simulink model "six_plus_six_AcmsteeringV09_main"  (R2014a)
settings: Solver=FixedStepDiscrete  StartTime=0.0  StopTime=10.0  FixedStep=0.0005  RelTol=1e-3
InitFcn:
  | Veh_Par_wxt
values from neighbouring files (symbols this model uses):
  acc_spdctl = [0 100]    [Veh_Par_wxt.m]
  ag_thr = ecucoder_cal(ag_thr)    [Veh_Par_wxt.m]
  B = 1.8    [Veh_Par_wxt.m]
  bra_em = 100    [Veh_Par_wxt.m]
  bra_pre_gz2 = 100/3    (= 33.3333333333)    [Veh_Par_wxt.m]
  bra_pre_gz34 = 10/3    (= 3.33333333333)    [Veh_Par_wxt.m]
  bra_pre_yd = 10/2    (= 5)    [Veh_Par_wxt.m]
  brakepre_dem_data = [0 1 2 3 4 5 6 7 8 9 10]    [Veh_Par_wxt.m]
  brakeTrq_dem_data = [0 125 251 376 502 627 753 878 1004 1129 1255]    [Veh_Par_wxt.m]
  bratrq_max = 4*1255    (= 5020)    [Veh_Par_wxt.m]
  eff_tran = 0.9    [Veh_Par_wxt.m]
  ESP_switch = ecucoder_cal(ESP_switch)    [Veh_Par_wxt.m]
  G = Mass*g    (= 15696)    [Veh_Par_wxt.m]
  kd1 = ecucoder_cal(kd1)    [Veh_Par_wxt.m]
  kd2 = 0    [Veh_Par_wxt.m]
  ki1 = ecucoder_cal(ki1)    [Veh_Par_wxt.m]
  ki2 = 1    [Veh_Par_wxt.m]
  kp1 = ecucoder_cal(kp1)    [Veh_Par_wxt.m]
  kp2 = 300    [Veh_Par_wxt.m]
  L = L1+L2    (= 2.9)    [Veh_Par_wxt.m]
  premax = 100    [Veh_Par_wxt.m]
  Radius = 0.4572/2    (= 0.2286)    [Veh_Par_wxt.m]
  RC_switch = ecucoder_cal(RC_switch)    [Veh_Par_wxt.m]
  s_opt_yi = 0.15    [Veh_Par_wxt.m]
  s_opt_zhuan = 0.8    [Veh_Par_wxt.m]
  s_opt_zhuan_add = 0.05    [Veh_Par_wxt.m]
  s_opt_zhuan_table = [0.8 0.8 0.3 0.3]    [Veh_Par_wxt.m]
  spd_map_mot = [0 499.85 999.79 1500 2000 2500 3000 3500 4000 4500 4999.8 5999.8]    [Veh_Par_wxt.m]
  spd_spdctl = [0 500]    [Veh_Par_wxt.m]
  speed_thr_park = 5/3.6/Radius*tras_ratio*30/pi    (= 464.143899364)    [Veh_Par_wxt.m]
  TCS_switch = ecucoder_cal(TCS_switch)    [Veh_Par_wxt.m]
  tras_ratio = 8    [Veh_Par_wxt.m]
  trq_map_mot = [70.5 70.012 71.154 65.797 53.917 45.159 38.073 32.685 27.48 17.133 14.949 10.07]    [Veh_Par_wxt.m]
  trqmax_yd = 70.5    [Veh_Par_wxt.m]
  trqmax_zx = 70.5    [Veh_Par_wxt.m]
  trqmaxneg = -70.5    [Veh_Par_wxt.m]
  v_gain = 0.9    [Veh_Par_wxt.m]
  v_table = [0 5 20 100]    [Veh_Par_wxt.m]
  v_thr_park = 5    [Veh_Par_wxt.m]
  zhidong_bianmazhi = [-140000 750000]    [Veh_Par_wxt.m]
  zhidong_down = -140000    [Veh_Par_wxt.m]
  zhidong_up = 750000    [Veh_Par_wxt.m]
  zhidong_youmen = [0 100]    [Veh_Par_wxt.m]
  zhuanxiang_bianmazhi = [-400000 0 400000]    [Veh_Par_wxt.m]
  zhuanxiang_down = -400000    [Veh_Par_wxt.m]
  zhuanxiang_up = 400000    [Veh_Par_wxt.m]
  zhuanxiang_youmen = [-100 0 100]    [Veh_Par_wxt.m]
undefined symbols (not defined in the file or in its folder): ecucoder_acal, guzhang_lf, guzhang_lm, guzhang_lr, guzhang_rf, guzhang_rm, guzhang_rr, myFIS
libraries: simulink x979, ec5744lib x59, fuzblock x2
(part 17 of 26)

== system six_plus_six_AcmsteeringV09_main/Data_input/MCU0_3/MCU0/MCU0_HighVol_Sub ==
  In1 : Inport
  Out1 : Outport
  wires:
  In1/1 -> Out1/1

== system six_plus_six_AcmsteeringV09_main/Data_input/MCU0_3/MCU0/MCU0_LiftCnt_Sub ==
  In1 : Inport
  Out1 : Outport
  wires:
  In1/1 -> Out1/1

== system six_plus_six_AcmsteeringV09_main/Data_input/MCU0_3/MCU0/MCU0_ShutDowAllow_Sub ==
  In1 : Inport
  Out1 : Outport
  wires:
  In1/1 -> Out1/1

== system six_plus_six_AcmsteeringV09_main/Data_input/MCU0_3/MCU0/MCU0_SpeedFdk_Sub ==
  In1 : Inport
  Out1 : Outport
  wires:
  In1/1 -> Out1/1

== system six_plus_six_AcmsteeringV09_main/Data_input/MCU0_3/MCU0/MCU0_TorqueFdk_Sub ==
  In1 : Inport
  Out1 : Outport
  wires:
  In1/1 -> Out1/1

== system six_plus_six_AcmsteeringV09_main/Data_input/MCU0_3/MCU0/MCU0_TorqueMax_Sub ==
  In1 : Inport
  Out1 : Outport
  wires:
  In1/1 -> Out1/1

== system six_plus_six_AcmsteeringV09_main/Data_input/MCU0_3/MCU0/MCU0_WorkStatus_Sub ==
  In1 : Inport
  Out1 : Outport
  wires:
  In1/1 -> Out1/1

== system six_plus_six_AcmsteeringV09_main/Data_input/MCU0_4/MCU0/MCU0_ControlMode_Sub ==
  In1 : Inport
  Out1 : Outport
  wires:
  In1/1 -> Out1/1

== system six_plus_six_AcmsteeringV09_main/Data_input/MCU0_4/MCU0/MCU0_EmergShutDown_Sub ==
  In1 : Inport
  Out1 : Outport
  wires:
  In1/1 -> Out1/1

== system six_plus_six_AcmsteeringV09_main/Data_input/MCU0_4/MCU0/MCU0_GearStatus_Sub ==
  In1 : Inport
  Out1 : Outport
  wires:
  In1/1 -> Out1/1

== system six_plus_six_AcmsteeringV09_main/Data_input/MCU0_4/MCU0/MCU0_HighVol_Sub ==
  In1 : Inport
  Out1 : Outport
  wires:
  In1/1 -> Out1/1

== system six_plus_six_AcmsteeringV09_main/Data_input/MCU0_4/MCU0/MCU0_LiftCnt_Sub ==
  In1 : Inport
  Out1 : Outport
  wires:
  In1/1 -> Out1/1

== system six_plus_six_AcmsteeringV09_main/Data_input/MCU0_4/MCU0/MCU0_ShutDowAllow_Sub ==
  In1 : Inport
  Out1 : Outport
  wires:
  In1/1 -> Out1/1

== system six_plus_six_AcmsteeringV09_main/Data_input/MCU0_4/MCU0/MCU0_SpeedFdk_Sub ==
  In1 : Inport
  Out1 : Outport
  wires:
  In1/1 -> Out1/1

== system six_plus_six_AcmsteeringV09_main/Data_input/MCU0_4/MCU0/MCU0_TorqueFdk_Sub ==
  In1 : Inport
  Out1 : Outport
  wires:
  In1/1 -> Out1/1

== system six_plus_six_AcmsteeringV09_main/Data_input/MCU0_4/MCU0/MCU0_TorqueMax_Sub ==
  In1 : Inport
  Out1 : Outport
  wires:
  In1/1 -> Out1/1

== system six_plus_six_AcmsteeringV09_main/Data_input/MCU0_4/MCU0/MCU0_WorkStatus_Sub ==
  In1 : Inport
  Out1 : Outport
  wires:
  In1/1 -> Out1/1

== system six_plus_six_AcmsteeringV09_main/Data_input/MCU0_5/MCU0/MCU0_ControlMode_Sub ==
  In1 : Inport
  Out1 : Outport
  wires:
  In1/1 -> Out1/1

== system six_plus_six_AcmsteeringV09_main/Data_input/MCU0_5/MCU0/MCU0_EmergShutDown_Sub ==
  In1 : Inport
  Out1 : Outport
  wires:
  In1/1 -> Out1/1

== system six_plus_six_AcmsteeringV09_main/Data_input/MCU0_5/MCU0/MCU0_GearStatus_Sub ==
  In1 : Inport
  Out1 : Outport
  wires:
  In1/1 -> Out1/1

== system six_plus_six_AcmsteeringV09_main/Data_input/MCU0_5/MCU0/MCU0_HighVol_Sub ==
  In1 : Inport
  Out1 : Outport
  wires:
  In1/1 -> Out1/1

== system six_plus_six_AcmsteeringV09_main/Data_input/MCU0_5/MCU0/MCU0_LiftCnt_Sub ==
  In1 : Inport
  Out1 : Outport
  wires:
  In1/1 -> Out1/1

== system six_plus_six_AcmsteeringV09_main/Data_input/MCU0_5/MCU0/MCU0_ShutDowAllow_Sub ==
  In1 : Inport
  Out1 : Outport
  wires:
  In1/1 -> Out1/1

== system six_plus_six_AcmsteeringV09_main/Data_input/MCU0_5/MCU0/MCU0_SpeedFdk_Sub ==
  In1 : Inport
  Out1 : Outport
  wires:
  In1/1 -> Out1/1

== system six_plus_six_AcmsteeringV09_main/Data_input/MCU0_5/MCU0/MCU0_TorqueFdk_Sub ==
  In1 : Inport
  Out1 : Outport
  wires:
  In1/1 -> Out1/1

== system six_plus_six_AcmsteeringV09_main/Data_input/MCU0_5/MCU0/MCU0_TorqueMax_Sub ==
  In1 : Inport
  Out1 : Outport
  wires:
  In1/1 -> Out1/1

== system six_plus_six_AcmsteeringV09_main/Data_input/MCU0_5/MCU0/MCU0_WorkStatus_Sub ==
  In1 : Inport
  Out1 : Outport
  wires:
  In1/1 -> Out1/1

== system six_plus_six_AcmsteeringV09_main/Data_input/MCU1/MCU1/MCU1_ControlTemp_Sub ==
  In1 : Inport
  Out1 : Outport
  wires:
  In1/1 -> Out1/1

== system six_plus_six_AcmsteeringV09_main/Data_input/MCU1/MCU1/MCU1_Idc_Sub ==
  In1 : Inport
  Out1 : Outport
  wires:
  In1/1 -> Out1/1

== system six_plus_six_AcmsteeringV09_main/Data_input/MCU1/MCU1/MCU1_MotorTemp_Sub ==
  In1 : Inport
  Out1 : Outport
  wires:
  In1/1 -> Out1/1

== system six_plus_six_AcmsteeringV09_main/Data_input/MCU1/MCU1/MCU1_PowerFdk_Sub ==
  In1 : Inport
  Out1 : Outport
  wires:
  In1/1 -> Out1/1

== system six_plus_six_AcmsteeringV09_main/Data_input/MCU1/MCU1/MCU1_Udc_Sub ==
  In1 : Inport
  Out1 : Outport
  wires:
  In1/1 -> Out1/1

== system six_plus_six_AcmsteeringV09_main/Data_input/MCU1_1/MCU1/MCU1_ControlTemp_Sub ==
  In1 : Inport
  Out1 : Outport
  wires:
  In1/1 -> Out1/1

== system six_plus_six_AcmsteeringV09_main/Data_input/MCU1_1/MCU1/MCU1_Idc_Sub ==
  In1 : Inport
  Out1 : Outport
  wires:
  In1/1 -> Out1/1

== system six_plus_six_AcmsteeringV09_main/Data_input/MCU1_1/MCU1/MCU1_MotorTemp_Sub ==
  In1 : Inport
  Out1 : Outport
  wires:
  In1/1 -> Out1/1

== system six_plus_six_AcmsteeringV09_main/Data_input/MCU1_1/MCU1/MCU1_PowerFdk_Sub ==
  In1 : Inport
  Out1 : Outport
  wires:
  In1/1 -> Out1/1

== system six_plus_six_AcmsteeringV09_main/Data_input/MCU1_1/MCU1/MCU1_Udc_Sub ==
  In1 : Inport
  Out1 : Outport
  wires:
  In1/1 -> Out1/1

== system six_plus_six_AcmsteeringV09_main/Data_input/MCU1_2/MCU1/MCU1_ControlTemp_Sub ==
  In1 : Inport
  Out1 : Outport
  wires:
  In1/1 -> Out1/1

== system six_plus_six_AcmsteeringV09_main/Data_input/MCU1_2/MCU1/MCU1_Idc_Sub ==
  In1 : Inport
  Out1 : Outport
  wires:
  In1/1 -> Out1/1

== system six_plus_six_AcmsteeringV09_main/Data_input/MCU1_2/MCU1/MCU1_MotorTemp_Sub ==
  In1 : Inport
  Out1 : Outport
  wires:
  In1/1 -> Out1/1

== system six_plus_six_AcmsteeringV09_main/Data_input/MCU1_2/MCU1/MCU1_PowerFdk_Sub ==
  In1 : Inport
  Out1 : Outport
  wires:
  In1/1 -> Out1/1

== system six_plus_six_AcmsteeringV09_main/Data_input/MCU1_2/MCU1/MCU1_Udc_Sub ==
  In1 : Inport
  Out1 : Outport
  wires:
  In1/1 -> Out1/1

== system six_plus_six_AcmsteeringV09_main/Data_input/MCU1_3/MCU1/MCU1_ControlTemp_Sub ==
  In1 : Inport
  Out1 : Outport
  wires:
  In1/1 -> Out1/1

== system six_plus_six_AcmsteeringV09_main/Data_input/MCU1_3/MCU1/MCU1_Idc_Sub ==
  In1 : Inport
  Out1 : Outport
  wires:
  In1/1 -> Out1/1

== system six_plus_six_AcmsteeringV09_main/Data_input/MCU1_3/MCU1/MCU1_MotorTemp_Sub ==
  In1 : Inport
  Out1 : Outport
  wires:
  In1/1 -> Out1/1

== system six_plus_six_AcmsteeringV09_main/Data_input/MCU1_3/MCU1/MCU1_PowerFdk_Sub ==
  In1 : Inport
  Out1 : Outport
  wires:
  In1/1 -> Out1/1

== system six_plus_six_AcmsteeringV09_main/Data_input/MCU1_3/MCU1/MCU1_Udc_Sub ==
  In1 : Inport
  Out1 : Outport
  wires:
  In1/1 -> Out1/1

== system six_plus_six_AcmsteeringV09_main/Data_input/MCU1_4/MCU1/MCU1_ControlTemp_Sub ==
  In1 : Inport
  Out1 : Outport
  wires:
  In1/1 -> Out1/1

== system six_plus_six_AcmsteeringV09_main/Data_input/MCU1_4/MCU1/MCU1_Idc_Sub ==
  In1 : Inport
  Out1 : Outport
  wires:
  In1/1 -> Out1/1

== system six_plus_six_AcmsteeringV09_main/Data_input/MCU1_4/MCU1/MCU1_MotorTemp_Sub ==
  In1 : Inport
  Out1 : Outport
  wires:
  In1/1 -> Out1/1

== system six_plus_six_AcmsteeringV09_main/Data_input/MCU1_4/MCU1/MCU1_PowerFdk_Sub ==
  In1 : Inport
  Out1 : Outport
  wires:
  In1/1 -> Out1/1

== system six_plus_six_AcmsteeringV09_main/Data_input/MCU1_4/MCU1/MCU1_Udc_Sub ==
  In1 : Inport
  Out1 : Outport
  wires:
  In1/1 -> Out1/1

== system six_plus_six_AcmsteeringV09_main/Data_input/MCU1_5/MCU1/MCU1_ControlTemp_Sub ==
  In1 : Inport
  Out1 : Outport
  wires:
  In1/1 -> Out1/1

== system six_plus_six_AcmsteeringV09_main/Data_input/MCU1_5/MCU1/MCU1_Idc_Sub ==
  In1 : Inport
  Out1 : Outport
  wires:
  In1/1 -> Out1/1

== system six_plus_six_AcmsteeringV09_main/Data_input/MCU1_5/MCU1/MCU1_MotorTemp_Sub ==
  In1 : Inport
  Out1 : Outport
  wires:
  In1/1 -> Out1/1

== system six_plus_six_AcmsteeringV09_main/Data_input/MCU1_5/MCU1/MCU1_PowerFdk_Sub ==
  In1 : Inport
  Out1 : Outport
  wires:
  In1/1 -> Out1/1

== system six_plus_six_AcmsteeringV09_main/Data_input/MCU1_5/MCU1/MCU1_Udc_Sub ==
  In1 : Inport
  Out1 : Outport
  wires:
  In1/1 -> Out1/1

== system six_plus_six_AcmsteeringV09_main/Data_input/MCU2/MCU2/MCU2_ActieDischargingFault_Sub ==
  In1 : Inport
  Out1 : Outport
  wires:
  In1/1 -> Out1/1

== system six_plus_six_AcmsteeringV09_main/Data_input/MCU2/MCU2/MCU2_CanCommunicationFault_Sub ==
  In1 : Inport
  Out1 : Outport
  wires:
  In1/1 -> Out1/1

== system six_plus_six_AcmsteeringV09_main/Data_input/MCU2/MCU2/MCU2_ControllerOverTemp_Sub ==
  In1 : Inport
  Out1 : Outport
  wires:
  In1/1 -> Out1/1

== system six_plus_six_AcmsteeringV09_main/Data_input/MCU2/MCU2/MCU2_ControllerOverload_Sub ==
  In1 : Inport
  Out1 : Outport
  wires:
  In1/1 -> Out1/1

== system six_plus_six_AcmsteeringV09_main/Data_input/MCU2/MCU2/MCU2_DownratingFault_Sub ==
  In1 : Inport
  Out1 : Outport
  wires:
  In1/1 -> Out1/1

== system six_plus_six_AcmsteeringV09_main/Data_input/MCU2/MCU2/MCU2_FaultLevel_Sub ==
  In1 : Inport
  Out1 : Outport
  wires:
  In1/1 -> Out1/1

== system six_plus_six_AcmsteeringV09_main/Data_input/MCU2/MCU2/MCU2_IGBTFault_Sub ==
  In1 : Inport
  Out1 : Outport
  wires:
  In1/1 -> Out1/1

== system six_plus_six_AcmsteeringV09_main/Data_input/MCU2/MCU2/MCU2_IdcSensorFault_Sub ==
  In1 : Inport
  Out1 : Outport
  wires:
  In1/1 -> Out1/1

== system six_plus_six_AcmsteeringV09_main/Data_input/MCU2/MCU2/MCU2_IuSensorFault_Sub ==
  In1 : Inport
  Out1 : Outport
  wires:
  In1/1 -> Out1/1

== system six_plus_six_AcmsteeringV09_main/Data_input/MCU2/MCU2/MCU2_IvSensorFault_Sub ==
  In1 : Inport
  Out1 : Outport
  wires:
  In1/1 -> Out1/1

== system six_plus_six_AcmsteeringV09_main/Data_input/MCU2/MCU2/MCU2_MemoryFault_Sub ==
  In1 : Inport
  Out1 : Outport
  wires:
  In1/1 -> Out1/1

== system six_plus_six_AcmsteeringV09_main/Data_input/MCU2/MCU2/MCU2_MotorOverLoad_Sub ==
  In1 : Inport
  Out1 : Outport
  wires:
  In1/1 -> Out1/1

== system six_plus_six_AcmsteeringV09_main/Data_input/MCU2/MCU2/MCU2_MotorOverSpeed_Sub ==
  In1 : Inport
  Out1 : Outport
  wires:
  In1/1 -> Out1/1

== system six_plus_six_AcmsteeringV09_main/Data_input/MCU2/MCU2/MCU2_MotorOverTemp_Sub ==
  In1 : Inport
  Out1 : Outport
  wires:
  In1/1 -> Out1/1

== system six_plus_six_AcmsteeringV09_main/Data_input/MCU2/MCU2/MCU2_MotorStallingFault_Sub ==
  In1 : Inport
  Out1 : Outport
  wires:
  In1/1 -> Out1/1

== system six_plus_six_AcmsteeringV09_main/Data_input/MCU2/MCU2/MCU2_OverVoltage_Sub ==
  In1 : Inport
  Out1 : Outport
  wires:
  In1/1 -> Out1/1

== system six_plus_six_AcmsteeringV09_main/Data_input/MCU2/MCU2/MCU2_RotaryInverterFault_Sub ==
  In1 : Inport
  Out1 : Outport
  wires:
  In1/1 -> Out1/1

== system six_plus_six_AcmsteeringV09_main/Data_input/MCU2/MCU2/MCU2_TempSensorFault_Sub ==
  In1 : Inport
  Out1 : Outport
  wires:
  In1/1 -> Out1/1

== system six_plus_six_AcmsteeringV09_main/Data_input/MCU2/MCU2/MCU2_UdcDetectionFault_Sub ==
  In1 : Inport
  Out1 : Outport
  wires:
  In1/1 -> Out1/1

== system six_plus_six_AcmsteeringV09_main/Data_input/MCU2/MCU2/MCU2_UnderVoltage_Sub ==
  In1 : Inport
  Out1 : Outport
  wires:
  In1/1 -> Out1/1

== system six_plus_six_AcmsteeringV09_main/Data_input/MCU2_1/MCU2/MCU2_ActieDischargingFault_Sub ==
  In1 : Inport
  Out1 : Outport
  wires:
  In1/1 -> Out1/1

== system six_plus_six_AcmsteeringV09_main/Data_input/MCU2_1/MCU2/MCU2_CanCommunicationFault_Sub ==
  In1 : Inport
  Out1 : Outport
  wires:
  In1/1 -> Out1/1

== system six_plus_six_AcmsteeringV09_main/Data_input/MCU2_1/MCU2/MCU2_ControllerOverTemp_Sub ==
  In1 : Inport
  Out1 : Outport
  wires:
  In1/1 -> Out1/1

== system six_plus_six_AcmsteeringV09_main/Data_input/MCU2_1/MCU2/MCU2_ControllerOverload_Sub ==
  In1 : Inport
  Out1 : Outport
  wires:
  In1/1 -> Out1/1

== system six_plus_six_AcmsteeringV09_main/Data_input/MCU2_1/MCU2/MCU2_DownratingFault_Sub ==
  In1 : Inport
  Out1 : Outport
  wires:
  In1/1 -> Out1/1

== system six_plus_six_AcmsteeringV09_main/Data_input/MCU2_1/MCU2/MCU2_FaultLevel_Sub ==
  In1 : Inport
  Out1 : Outport
  wires:
  In1/1 -> Out1/1

== system six_plus_six_AcmsteeringV09_main/Data_input/MCU2_1/MCU2/MCU2_IGBTFault_Sub ==
  In1 : Inport
  Out1 : Outport
  wires:
  In1/1 -> Out1/1

== system six_plus_six_AcmsteeringV09_main/Data_input/MCU2_1/MCU2/MCU2_IdcSensorFault_Sub ==
  In1 : Inport
  Out1 : Outport
  wires:
  In1/1 -> Out1/1

== system six_plus_six_AcmsteeringV09_main/Data_input/MCU2_1/MCU2/MCU2_IuSensorFault_Sub ==
  In1 : Inport
  Out1 : Outport
  wires:
  In1/1 -> Out1/1

== system six_plus_six_AcmsteeringV09_main/Data_input/MCU2_1/MCU2/MCU2_IvSensorFault_Sub ==
  In1 : Inport
  Out1 : Outport
  wires:
  In1/1 -> Out1/1

== system six_plus_six_AcmsteeringV09_main/Data_input/MCU2_1/MCU2/MCU2_MemoryFault_Sub ==
  In1 : Inport
  Out1 : Outport
  wires:
  In1/1 -> Out1/1

== system six_plus_six_AcmsteeringV09_main/Data_input/MCU2_1/MCU2/MCU2_MotorOverLoad_Sub ==
  In1 : Inport
  Out1 : Outport
  wires:
  In1/1 -> Out1/1

== system six_plus_six_AcmsteeringV09_main/Data_input/MCU2_1/MCU2/MCU2_MotorOverSpeed_Sub ==
  In1 : Inport
  Out1 : Outport
  wires:
  In1/1 -> Out1/1

== system six_plus_six_AcmsteeringV09_main/Data_input/MCU2_1/MCU2/MCU2_MotorOverTemp_Sub ==
  In1 : Inport
  Out1 : Outport
  wires:
  In1/1 -> Out1/1

== system six_plus_six_AcmsteeringV09_main/Data_input/MCU2_1/MCU2/MCU2_MotorStallingFault_Sub ==
  In1 : Inport
  Out1 : Outport
  wires:
  In1/1 -> Out1/1

== system six_plus_six_AcmsteeringV09_main/Data_input/MCU2_1/MCU2/MCU2_OverVoltage_Sub ==
  In1 : Inport
  Out1 : Outport
  wires:
  In1/1 -> Out1/1

== system six_plus_six_AcmsteeringV09_main/Data_input/MCU2_1/MCU2/MCU2_RotaryInverterFault_Sub ==
  In1 : Inport
  Out1 : Outport
  wires:
  In1/1 -> Out1/1

== system six_plus_six_AcmsteeringV09_main/Data_input/MCU2_1/MCU2/MCU2_TempSensorFault_Sub ==
  In1 : Inport
  Out1 : Outport
  wires:
  In1/1 -> Out1/1

== system six_plus_six_AcmsteeringV09_main/Data_input/MCU2_1/MCU2/MCU2_UdcDetectionFault_Sub ==
  In1 : Inport
  Out1 : Outport
  wires:
  In1/1 -> Out1/1

== system six_plus_six_AcmsteeringV09_main/Data_input/MCU2_1/MCU2/MCU2_UnderVoltage_Sub ==
  In1 : Inport
  Out1 : Outport
  wires:
  In1/1 -> Out1/1

== system six_plus_six_AcmsteeringV09_main/Data_input/MCU2_2/MCU2/MCU2_ActieDischargingFault_Sub ==
  In1 : Inport
  Out1 : Outport
  wires:
  In1/1 -> Out1/1

== system six_plus_six_AcmsteeringV09_main/Data_input/MCU2_2/MCU2/MCU2_CanCommunicationFault_Sub ==
  In1 : Inport
  Out1 : Outport
  wires:
  In1/1 -> Out1/1

== system six_plus_six_AcmsteeringV09_main/Data_input/MCU2_2/MCU2/MCU2_ControllerOverTemp_Sub ==
  In1 : Inport
  Out1 : Outport
  wires:
  In1/1 -> Out1/1

== system six_plus_six_AcmsteeringV09_main/Data_input/MCU2_2/MCU2/MCU2_ControllerOverload_Sub ==
  In1 : Inport
  Out1 : Outport
  wires:
  In1/1 -> Out1/1

== system six_plus_six_AcmsteeringV09_main/Data_input/MCU2_2/MCU2/MCU2_DownratingFault_Sub ==
  In1 : Inport
  Out1 : Outport
  wires:
  In1/1 -> Out1/1

== system six_plus_six_AcmsteeringV09_main/Data_input/MCU2_2/MCU2/MCU2_FaultLevel_Sub ==
  In1 : Inport
  Out1 : Outport
  wires:
  In1/1 -> Out1/1

== system six_plus_six_AcmsteeringV09_main/Data_input/MCU2_2/MCU2/MCU2_IGBTFault_Sub ==
  In1 : Inport
  Out1 : Outport
  wires:
  In1/1 -> Out1/1

== system six_plus_six_AcmsteeringV09_main/Data_input/MCU2_2/MCU2/MCU2_IdcSensorFault_Sub ==
  In1 : Inport
  Out1 : Outport
  wires:
  In1/1 -> Out1/1

== system six_plus_six_AcmsteeringV09_main/Data_input/MCU2_2/MCU2/MCU2_IuSensorFault_Sub ==
  In1 : Inport
  Out1 : Outport
  wires:
  In1/1 -> Out1/1

== system six_plus_six_AcmsteeringV09_main/Data_input/MCU2_2/MCU2/MCU2_IvSensorFault_Sub ==
  In1 : Inport
  Out1 : Outport
  wires:
  In1/1 -> Out1/1

== system six_plus_six_AcmsteeringV09_main/Data_input/MCU2_2/MCU2/MCU2_MemoryFault_Sub ==
  In1 : Inport
  Out1 : Outport
  wires:
  In1/1 -> Out1/1

== system six_plus_six_AcmsteeringV09_main/Data_input/MCU2_2/MCU2/MCU2_MotorOverLoad_Sub ==
  In1 : Inport
  Out1 : Outport
  wires:
  In1/1 -> Out1/1

== system six_plus_six_AcmsteeringV09_main/Data_input/MCU2_2/MCU2/MCU2_MotorOverSpeed_Sub ==
  In1 : Inport
  Out1 : Outport
  wires:
  In1/1 -> Out1/1

== system six_plus_six_AcmsteeringV09_main/Data_input/MCU2_2/MCU2/MCU2_MotorOverTemp_Sub ==
  In1 : Inport
  Out1 : Outport
  wires:
  In1/1 -> Out1/1

== system six_plus_six_AcmsteeringV09_main/Data_input/MCU2_2/MCU2/MCU2_MotorStallingFault_Sub ==
  In1 : Inport
  Out1 : Outport
  wires:
  In1/1 -> Out1/1

== system six_plus_six_AcmsteeringV09_main/Data_input/MCU2_2/MCU2/MCU2_OverVoltage_Sub ==
  In1 : Inport
  Out1 : Outport
  wires:
  In1/1 -> Out1/1

== system six_plus_six_AcmsteeringV09_main/Data_input/MCU2_2/MCU2/MCU2_RotaryInverterFault_Sub ==
  In1 : Inport
  Out1 : Outport
  wires:
  In1/1 -> Out1/1

== system six_plus_six_AcmsteeringV09_main/Data_input/MCU2_2/MCU2/MCU2_TempSensorFault_Sub ==
  In1 : Inport
  Out1 : Outport
  wires:
  In1/1 -> Out1/1

== system six_plus_six_AcmsteeringV09_main/Data_input/MCU2_2/MCU2/MCU2_UdcDetectionFault_Sub ==
  In1 : Inport
  Out1 : Outport
  wires:
  In1/1 -> Out1/1

== system six_plus_six_AcmsteeringV09_main/Data_input/MCU2_2/MCU2/MCU2_UnderVoltage_Sub ==
  In1 : Inport
  Out1 : Outport
  wires:
  In1/1 -> Out1/1

== system six_plus_six_AcmsteeringV09_main/Data_input/MCU2_3/MCU2/MCU2_ActieDischargingFault_Sub ==
  In1 : Inport
  Out1 : Outport
  wires:
  In1/1 -> Out1/1

== system six_plus_six_AcmsteeringV09_main/Data_input/MCU2_3/MCU2/MCU2_CanCommunicationFault_Sub ==
  In1 : Inport
  Out1 : Outport
  wires:
  In1/1 -> Out1/1

== system six_plus_six_AcmsteeringV09_main/Data_input/MCU2_3/MCU2/MCU2_ControllerOverTemp_Sub ==
  In1 : Inport
  Out1 : Outport
  wires:
  In1/1 -> Out1/1

== system six_plus_six_AcmsteeringV09_main/Data_input/MCU2_3/MCU2/MCU2_ControllerOverload_Sub ==
  In1 : Inport
  Out1 : Outport
  wires:
  In1/1 -> Out1/1

== system six_plus_six_AcmsteeringV09_main/Data_input/MCU2_3/MCU2/MCU2_DownratingFault_Sub ==
  In1 : Inport
  Out1 : Outport
  wires:
  In1/1 -> Out1/1

== system six_plus_six_AcmsteeringV09_main/Data_input/MCU2_3/MCU2/MCU2_FaultLevel_Sub ==
  In1 : Inport
  Out1 : Outport
  wires:
  In1/1 -> Out1/1

== system six_plus_six_AcmsteeringV09_main/Data_input/MCU2_3/MCU2/MCU2_IGBTFault_Sub ==
  In1 : Inport
  Out1 : Outport
  wires:
  In1/1 -> Out1/1

== system six_plus_six_AcmsteeringV09_main/Data_input/MCU2_3/MCU2/MCU2_IdcSensorFault_Sub ==
  In1 : Inport
  Out1 : Outport
  wires:
  In1/1 -> Out1/1

== system six_plus_six_AcmsteeringV09_main/Data_input/MCU2_3/MCU2/MCU2_IuSensorFault_Sub ==
  In1 : Inport
  Out1 : Outport
  wires:
  In1/1 -> Out1/1

== system six_plus_six_AcmsteeringV09_main/Data_input/MCU2_3/MCU2/MCU2_IvSensorFault_Sub ==
  In1 : Inport
  Out1 : Outport
  wires:
  In1/1 -> Out1/1

== system six_plus_six_AcmsteeringV09_main/Data_input/MCU2_3/MCU2/MCU2_MemoryFault_Sub ==
  In1 : Inport
  Out1 : Outport
  wires:
  In1/1 -> Out1/1

== system six_plus_six_AcmsteeringV09_main/Data_input/MCU2_3/MCU2/MCU2_MotorOverLoad_Sub ==
  In1 : Inport
  Out1 : Outport
  wires:
  In1/1 -> Out1/1

== system six_plus_six_AcmsteeringV09_main/Data_input/MCU2_3/MCU2/MCU2_MotorOverSpeed_Sub ==
  In1 : Inport
  Out1 : Outport
  wires:
  In1/1 -> Out1/1

== system six_plus_six_AcmsteeringV09_main/Data_input/MCU2_3/MCU2/MCU2_MotorOverTemp_Sub ==
  In1 : Inport
  Out1 : Outport
  wires:
  In1/1 -> Out1/1

== system six_plus_six_AcmsteeringV09_main/Data_input/MCU2_3/MCU2/MCU2_MotorStallingFault_Sub ==
  In1 : Inport
  Out1 : Outport
  wires:
  In1/1 -> Out1/1

== system six_plus_six_AcmsteeringV09_main/Data_input/MCU2_3/MCU2/MCU2_OverVoltage_Sub ==
  In1 : Inport
  Out1 : Outport
  wires:
  In1/1 -> Out1/1

== system six_plus_six_AcmsteeringV09_main/Data_input/MCU2_3/MCU2/MCU2_RotaryInverterFault_Sub ==
  In1 : Inport
  Out1 : Outport
  wires:
  In1/1 -> Out1/1

== system six_plus_six_AcmsteeringV09_main/Data_input/MCU2_3/MCU2/MCU2_TempSensorFault_Sub ==
  In1 : Inport
  Out1 : Outport
  wires:
  In1/1 -> Out1/1

== system six_plus_six_AcmsteeringV09_main/Data_input/MCU2_3/MCU2/MCU2_UdcDetectionFault_Sub ==
  In1 : Inport
  Out1 : Outport
  wires:
  In1/1 -> Out1/1

== system six_plus_six_AcmsteeringV09_main/Data_input/MCU2_3/MCU2/MCU2_UnderVoltage_Sub ==
  In1 : Inport
  Out1 : Outport
  wires:
  In1/1 -> Out1/1

== system six_plus_six_AcmsteeringV09_main/Data_input/MCU2_4/MCU2/MCU2_ActieDischargingFault_Sub ==
  In1 : Inport
  Out1 : Outport
  wires:
  In1/1 -> Out1/1

== system six_plus_six_AcmsteeringV09_main/Data_input/MCU2_4/MCU2/MCU2_CanCommunicationFault_Sub ==
  In1 : Inport
  Out1 : Outport
  wires:
  In1/1 -> Out1/1

== system six_plus_six_AcmsteeringV09_main/Data_input/MCU2_4/MCU2/MCU2_ControllerOverTemp_Sub ==
  In1 : Inport
  Out1 : Outport
  wires:
  In1/1 -> Out1/1

== system six_plus_six_AcmsteeringV09_main/Data_input/MCU2_4/MCU2/MCU2_ControllerOverload_Sub ==
  In1 : Inport
  Out1 : Outport
  wires:
  In1/1 -> Out1/1

== system six_plus_six_AcmsteeringV09_main/Data_input/MCU2_4/MCU2/MCU2_DownratingFault_Sub ==
  In1 : Inport
  Out1 : Outport
  wires:
  In1/1 -> Out1/1

== system six_plus_six_AcmsteeringV09_main/Data_input/MCU2_4/MCU2/MCU2_FaultLevel_Sub ==
  In1 : Inport
  Out1 : Outport
  wires:
  In1/1 -> Out1/1

== system six_plus_six_AcmsteeringV09_main/Data_input/MCU2_4/MCU2/MCU2_IGBTFault_Sub ==
  In1 : Inport
  Out1 : Outport
  wires:
  In1/1 -> Out1/1

== system six_plus_six_AcmsteeringV09_main/Data_input/MCU2_4/MCU2/MCU2_IdcSensorFault_Sub ==
  In1 : Inport
  Out1 : Outport
  wires:
  In1/1 -> Out1/1

== system six_plus_six_AcmsteeringV09_main/Data_input/MCU2_4/MCU2/MCU2_IuSensorFault_Sub ==
  In1 : Inport
  Out1 : Outport
  wires:
  In1/1 -> Out1/1

== system six_plus_six_AcmsteeringV09_main/Data_input/MCU2_4/MCU2/MCU2_IvSensorFault_Sub ==
  In1 : Inport
  Out1 : Outport
  wires:
  In1/1 -> Out1/1

== system six_plus_six_AcmsteeringV09_main/Data_input/MCU2_4/MCU2/MCU2_MemoryFault_Sub ==
  In1 : Inport
  Out1 : Outport
  wires:
  In1/1 -> Out1/1

== system six_plus_six_AcmsteeringV09_main/Data_input/MCU2_4/MCU2/MCU2_MotorOverLoad_Sub ==
  In1 : Inport
  Out1 : Outport
  wires:
  In1/1 -> Out1/1

== system six_plus_six_AcmsteeringV09_main/Data_input/MCU2_4/MCU2/MCU2_MotorOverSpeed_Sub ==
  In1 : Inport
  Out1 : Outport
  wires:
  In1/1 -> Out1/1

== system six_plus_six_AcmsteeringV09_main/Data_input/MCU2_4/MCU2/MCU2_MotorOverTemp_Sub ==
  In1 : Inport
  Out1 : Outport
  wires:
  In1/1 -> Out1/1

== system six_plus_six_AcmsteeringV09_main/Data_input/MCU2_4/MCU2/MCU2_MotorStallingFault_Sub ==
  In1 : Inport
  Out1 : Outport
  wires:
  In1/1 -> Out1/1

== system six_plus_six_AcmsteeringV09_main/Data_input/MCU2_4/MCU2/MCU2_OverVoltage_Sub ==
  In1 : Inport
  Out1 : Outport
  wires:
  In1/1 -> Out1/1

== system six_plus_six_AcmsteeringV09_main/Data_input/MCU2_4/MCU2/MCU2_RotaryInverterFault_Sub ==
  In1 : Inport
  Out1 : Outport
  wires:
  In1/1 -> Out1/1

== system six_plus_six_AcmsteeringV09_main/Data_input/MCU2_4/MCU2/MCU2_TempSensorFault_Sub ==
  In1 : Inport
  Out1 : Outport
  wires:
  In1/1 -> Out1/1

== system six_plus_six_AcmsteeringV09_main/Data_input/MCU2_4/MCU2/MCU2_UdcDetectionFault_Sub ==
  In1 : Inport
  Out1 : Outport
  wires:
  In1/1 -> Out1/1

== system six_plus_six_AcmsteeringV09_main/Data_input/MCU2_4/MCU2/MCU2_UnderVoltage_Sub ==
  In1 : Inport
  Out1 : Outport
  wires:
  In1/1 -> Out1/1

== system six_plus_six_AcmsteeringV09_main/Data_input/MCU2_5/MCU2/MCU2_ActieDischargingFault_Sub ==
  In1 : Inport
  Out1 : Outport
  wires:
  In1/1 -> Out1/1

== system six_plus_six_AcmsteeringV09_main/Data_input/MCU2_5/MCU2/MCU2_CanCommunicationFault_Sub ==
  In1 : Inport
  Out1 : Outport
  wires:
  In1/1 -> Out1/1

== system six_plus_six_AcmsteeringV09_main/Data_input/MCU2_5/MCU2/MCU2_ControllerOverTemp_Sub ==
  In1 : Inport
  Out1 : Outport
  wires:
  In1/1 -> Out1/1

== system six_plus_six_AcmsteeringV09_main/Data_input/MCU2_5/MCU2/MCU2_ControllerOverload_Sub ==
  In1 : Inport
  Out1 : Outport
  wires:
  In1/1 -> Out1/1

== system six_plus_six_AcmsteeringV09_main/Data_input/MCU2_5/MCU2/MCU2_DownratingFault_Sub ==
  In1 : Inport
  Out1 : Outport
  wires:
  In1/1 -> Out1/1

== system six_plus_six_AcmsteeringV09_main/Data_input/MCU2_5/MCU2/MCU2_FaultLevel_Sub ==
  In1 : Inport
  Out1 : Outport
  wires:
  In1/1 -> Out1/1

== system six_plus_six_AcmsteeringV09_main/Data_input/MCU2_5/MCU2/MCU2_IGBTFault_Sub ==
  In1 : Inport
  Out1 : Outport
  wires:
  In1/1 -> Out1/1

== system six_plus_six_AcmsteeringV09_main/Data_input/MCU2_5/MCU2/MCU2_IdcSensorFault_Sub ==
  In1 : Inport
  Out1 : Outport
  wires:
  In1/1 -> Out1/1

== system six_plus_six_AcmsteeringV09_main/Data_input/MCU2_5/MCU2/MCU2_IuSensorFault_Sub ==
  In1 : Inport
  Out1 : Outport
  wires:
  In1/1 -> Out1/1

== system six_plus_six_AcmsteeringV09_main/Data_input/MCU2_5/MCU2/MCU2_IvSensorFault_Sub ==
  In1 : Inport
  Out1 : Outport
  wires:
  In1/1 -> Out1/1

== system six_plus_six_AcmsteeringV09_main/Data_input/MCU2_5/MCU2/MCU2_MemoryFault_Sub ==
  In1 : Inport
  Out1 : Outport
  wires:
  In1/1 -> Out1/1

== system six_plus_six_AcmsteeringV09_main/Data_input/MCU2_5/MCU2/MCU2_MotorOverLoad_Sub ==
  In1 : Inport
  Out1 : Outport
  wires:
  In1/1 -> Out1/1

== system six_plus_six_AcmsteeringV09_main/Data_input/MCU2_5/MCU2/MCU2_MotorOverSpeed_Sub ==
  In1 : Inport
  Out1 : Outport
  wires:
  In1/1 -> Out1/1

== system six_plus_six_AcmsteeringV09_main/Data_input/MCU2_5/MCU2/MCU2_MotorOverTemp_Sub ==
  In1 : Inport
  Out1 : Outport
  wires:
  In1/1 -> Out1/1

== system six_plus_six_AcmsteeringV09_main/Data_input/MCU2_5/MCU2/MCU2_MotorStallingFault_Sub ==
  In1 : Inport
  Out1 : Outport
  wires:
  In1/1 -> Out1/1

== system six_plus_six_AcmsteeringV09_main/Data_input/MCU2_5/MCU2/MCU2_OverVoltage_Sub ==
  In1 : Inport
  Out1 : Outport
  wires:
  In1/1 -> Out1/1

== system six_plus_six_AcmsteeringV09_main/Data_input/MCU2_5/MCU2/MCU2_RotaryInverterFault_Sub ==
  In1 : Inport
  Out1 : Outport
  wires:
  In1/1 -> Out1/1

== system six_plus_six_AcmsteeringV09_main/Data_input/MCU2_5/MCU2/MCU2_TempSensorFault_Sub ==
  In1 : Inport
  Out1 : Outport
  wires:
  In1/1 -> Out1/1

== system six_plus_six_AcmsteeringV09_main/Data_input/MCU2_5/MCU2/MCU2_UdcDetectionFault_Sub ==
  In1 : Inport
  Out1 : Outport
  wires:
  In1/1 -> Out1/1

== system six_plus_six_AcmsteeringV09_main/Data_input/MCU2_5/MCU2/MCU2_UnderVoltage_Sub ==
  In1 : Inport
  Out1 : Outport
  wires:
  In1/1 -> Out1/1

== system six_plus_six_AcmsteeringV09_main/Data_input/RemoteControl1/Yaokong2/LIFEspan_Sub ==
  In1 : Inport
  Out1 : Outport
  wires:
  In1/1 -> Out1/1

== system six_plus_six_AcmsteeringV09_main/Data_input/RemoteControl1/Yaokong2/SA_Sub ==
  In1 : Inport
  Out1 : Outport
  wires:
  In1/1 -> Out1/1

== system six_plus_six_AcmsteeringV09_main/Data_input/RemoteControl1/Yaokong2/SD_Sub ==
  In1 : Inport
  Out1 : Outport
  wires:
  In1/1 -> Out1/1

== system six_plus_six_AcmsteeringV09_main/Data_input/RemoteControl1/Yaokong2/SE_Sub ==
  In1 : Inport
  Out1 : Outport
  wires:
  In1/1 -> Out1/1

== system six_plus_six_AcmsteeringV09_main/Data_input/RemoteControl1/Yaokong2/SH_Sub ==
  In1 : Inport
  Out1 : Outport
  wires:
  In1/1 -> Out1/1

== system six_plus_six_AcmsteeringV09_main/Data_input/RemoteControl2/Yaokong1/Leftstick_leftright_Sub ==
  In1 : Inport
  Out1 : Outport
  wires:
  In1/1 -> Out1/1

== system six_plus_six_AcmsteeringV09_main/Data_input/RemoteControl2/Yaokong1/Leftstick_updown_Sub ==
  In1 : Inport
  Out1 : Outport
  wires:
  In1/1 -> Out1/1

== system six_plus_six_AcmsteeringV09_main/Data_input/RemoteControl2/Yaokong1/Rightstick_leftright_Sub ==
  In1 : Inport
  Out1 : Outport
  wires:
  In1/1 -> Out1/1

== system six_plus_six_AcmsteeringV09_main/Data_input/RemoteControl2/Yaokong1/Rightstick_updown_Sub ==
  In1 : Inport
  Out1 : Outport
  wires:
  In1/1 -> Out1/1

== system six_plus_six_AcmsteeringV09_main/MainControl/mode_control/Park/park ==
  Signals : Inport
  1-D Lookup Table1 : Lookup_n-D  NumberOfTableDimensions=1  BreakpointsForDimension1=zhuanxiang_youmen  Table=zhuanxiang_bianmazhi  InternalRulePriority=Speed  RndMeth=Simplest  InputSameDT=on
  1-D Lookup Table2 : Lookup_n-D  NumberOfTableDimensions=1  BreakpointsForDimension1=zhidong_youmen  Table=zhidong_bianmazhi  InternalRulePriority=Speed  RndMeth=Simplest  InputSameDT=on
  Add : Sum
  Bus Selector : BusSelector  OutputSignals=RemoteControl_dem.steer_dem,RemoteControl_dem.brake_dem
  Constant1 : Constant  Value=100000  OutDataTypeStr=single  SampleTime=-1
  Gain : Gain  Gain=0.5
  Gain1 : Gain  Gain=-1
  HeartBeat : MATLAB Function  TreatAsAtomicUnit=on
  HeartBeat1 : MATLAB Function  TreatAsAtomicUnit=on
  HeartBeat2 : MATLAB Function  TreatAsAtomicUnit=on
  HeartBeat3 : MATLAB Function  TreatAsAtomicUnit=on
  HeartBeat4 : MATLAB Function  TreatAsAtomicUnit=on
  HeartBeat5 : MATLAB Function  TreatAsAtomicUnit=on
  Memory{,1..4,6} (6 alike) : Memory  InheritSampleTime=on
  Mux{,1..5} (6 alike) : Mux  Inputs=6
  Saturation : Saturate  UpperLimit=zhuanxiang_up  LowerLimit=zhuanxiang_down
  Saturation1 : Saturate  UpperLimit=zhuanxiang_up  LowerLimit=zhuanxiang_down
  Saturation2 : Saturate  UpperLimit=zhuanxiang_up  LowerLimit=zhuanxiang_down
  Saturation3 : Saturate  UpperLimit=zhidong_up  LowerLimit=zhidong_down
  SpdSet_dem{,1..5} (6 alike) : Constant  Value=0  OutDataTypeStr=single  SampleTime=-1
  TrqSet_dem{,1..5} (6 alike) : Constant  Value=0  OutDataTypeStr=single  SampleTime=-1
  mot_enable{,1..5} (6 alike) : Constant  Value=0  OutDataTypeStr=single  SampleTime=-1
  mot_gear{,1..5} (6 alike) : Constant  Value=0  OutDataTypeStr=single  SampleTime=-1
  mot_mode{,1..5} (6 alike) : Constant  Value=0  OutDataTypeStr=single  SampleTime=-1
  mot_lf : Outport
  mot_lm : Outport  Port=2
  mot_lr : Outport  Port=3
  mot_rf : Outport  Port=4
  mot_rm : Outport  Port=5
  mot_rr : Outport  Port=6
  motec_position_1 : Outport  Port=7
  motec_position_2 : Outport  Port=8
  motec_position_3 : Outport  Port=9
  motec_position_4 : Outport  Port=10
  wires:
  mot_gear/1 -> Mux/3
  mot_mode/1 -> Mux/2
  SpdSet_dem/1 -> Mux/4
  TrqSet_dem/1 -> Mux/5
  Mux/1 -> mot_lf/1
  HeartBeat/1(life) -> Mux/6, Memory/1
  Memory/1 -> HeartBeat/1(life_pre)
  Add/1 -> Saturation3/1
  mot_enable/1 -> Mux/1
  mot_gear1/1 -> Mux2/3
  mot_mode2/1 -> Mux2/2
  SpdSet_dem1/1 -> Mux2/4
  TrqSet_dem1/1 -> Mux2/5
  Mux2/1 -> mot_rf/1
  HeartBeat2/1(life) -> Memory2/1, Mux2/6
  Memory2/1 -> HeartBeat2/1(life_pre)
  mot_enable1/1 -> Mux2/1
  mot_gear2/1 -> Mux4/3
  mot_mode4/1 -> Mux4/2
  SpdSet_dem4/1 -> Mux4/4
  TrqSet_dem4/1 -> Mux4/5
  Mux4/1 -> mot_lm/1
  HeartBeat3/1(life) -> Memory4/1, Mux4/6
  Memory4/1 -> HeartBeat3/1(life_pre)
  mot_enable3/1 -> Mux4/1
  mot_gear3/1 -> Mux5/3
  mot_mode5/1 -> Mux5/2
  SpdSet_dem5/1 -> Mux5/4
  TrqSet_dem5/1 -> Mux5/5
  Mux5/1 -> mot_rm/1
  HeartBeat4/1(life) -> Mux5/6, Memory6/1
  Memory6/1 -> HeartBeat4/1(life_pre)
  mot_enable5/1 -> Mux5/1
  mot_gear4/1 -> Mux1/3
  mot_mode1/1 -> Mux1/2
  SpdSet_dem2/1 -> Mux1/4
  TrqSet_dem2/1 -> Mux1/5
  Mux1/1 -> mot_lr/1
  HeartBeat1/1(life) -> Memory1/1, Mux1/6
  Memory1/1 -> HeartBeat1/1(life_pre)
  mot_enable4/1 -> Mux1/1
  mot_gear5/1 -> Mux3/3
  mot_mode3/1 -> Mux3/2
  SpdSet_dem3/1 -> Mux3/4
  TrqSet_dem3/1 -> Mux3/5
  Mux3/1 -> mot_rr/1
  HeartBeat5/1(life) -> Memory3/1, Mux3/6
  Memory3/1 -> HeartBeat5/1(life_pre)
  mot_enable2/1 -> Mux3/1
  1-D Lookup Table1/1 -> Gain1/1, Gain/1, Saturation/1
  Signals/1 -> Bus Selector/1
  Gain1/1 -> Saturation2/1
  Bus Selector/1 -> 1-D Lookup Table1/1  "<steer_dem>"
  Gain/1 -> Saturation1/1
  Saturation/1 -> motec_position_1/1
  Saturation1/1 -> motec_position_2/1
  Saturation2/1 -> motec_position_3/1
  Saturation3/1 -> motec_position_4/1
  1-D Lookup Table2/1 -> Add/1
  Bus Selector/2 -> 1-D Lookup Table2/1  "<brake_dem>"
  Constant1/1 -> Add/2

== system six_plus_six_AcmsteeringV09_main/MainControl/mode_control/backward/backward ==
  Signals : Inport
  Brake : Subsystem  TreatAsAtomicUnit=on
  Bus Selector : BusSelector  OutputSignals=RemoteControl_dem.acc_dem,RemoteControl_dem.brake_dem,RemoteControl_dem.HAC
  Drive : Subsystem  TreatAsAtomicUnit=on
  MATLAB Function : MATLAB Function  TreatAsAtomicUnit=on
  Multiport Switch : MultiPortSwitch  DataPortOrder=Zero-based contiguous  Inputs=2
  Switch Case1 : SwitchCase  CaseConditions={0,1}  ShowDefaultCase=off
  backward_dem : Outport
  wires:
  Signals/1 -> Brake/1(Signals), Drive/1(Signals), Bus Selector/1
  Multiport Switch/1 -> backward_dem/1
  Switch Case1/1 -> Drive/Action
  Switch Case1/2 -> Brake/Action
  Bus Selector/1 -> MATLAB Function/1(acc_dem)  "<acc_dem>"
  MATLAB Function/1(y) -> Multiport Switch/1, Switch Case1/1
  Drive/1(backward_dem) -> Multiport Switch/2
  Brake/1(backward_dem) -> Multiport Switch/3
  Bus Selector/2 -> MATLAB Function/2(brake_dem)  "<brake_dem>"
  Bus Selector/3 -> MATLAB Function/3(HAC)  "<HAC>"

== system six_plus_six_AcmsteeringV09_main/MainControl/mode_control/center_steer/center_steer ==
  Signals : Inport
  1-D Lookup Table1 : Lookup_n-D  NumberOfTableDimensions=1  BreakpointsForDimension1=brakeTrq_dem_data  Table=brakepre_dem_data  InternalRulePriority=Speed  RndMeth=Simplest  InputSameDT=on
  1-D Lookup Table2 : Lookup_n-D  NumberOfTableDimensions=1  BreakpointsForDimension1=zhidong_youmen  Table=zhidong_bianmazhi  InternalRulePriority=Speed  RndMeth=Simplest  InputSameDT=on
  1-D Lookup Table3 : Lookup_n-D  NumberOfTableDimensions=1  BreakpointsForDimension1=brakeTrq_dem_data  Table=brakepre_dem_data  InternalRulePriority=Speed  RndMeth=Simplest  InputSameDT=on
  Abs{,1..5} (6 alike) : Abs  OutDataTypeStr=single
  Bus Selector : BusSelector  OutputSignals=RemoteControl_dem.brake_dem
  Bus Selector5 : BusSelector  OutputSignals=RemoteControl_dem.steer_dem,CCM.CCM1.BMS5.BMS5_15s_InstanceDisPower,CCM.CCM2.BMS5_1.BMS5_1_15s_InstanceDisPower,CCM.CCM3.BMS5_2.BMS5_2_15s_InstanceDisPower,MOTOR.MOTOR1.MCU0.MCU0_SpeedFdk,MOTOR.MOTOR3.MCU0_2.MCU0_2SpeedFdk,MOTOR.MOTOR5.MCU0_4.MCU0_4SpeedFdk,MOTOR.MOTOR2.MCU0_1.MCU0_1SpeedFdk,MOTOR.MOTOR4.MCU0_3.MCU0_3SpeedFdk,MOTOR.MOTOR6.MCU0_5.MCU0_5SpeedFdk,MOTOR.MOTOR1.MCU0.MCU0_TorqueMax,MOTOR.MOTOR3.MCU0_2.MCU0_2TorqueMax,MOTOR.MOTOR5.MCU0_4.MCU0_4TorqueMax,MOTOR.MOTOR2.MCU0_1.MCU0_1TorqueMax,MOTOR.MOTOR4.MCU0_3.MCU0_3TorqueMax,MOTOR.MOTOR6.MCU0_5.MCU0_5TorqueMax
  Bus Selector7 : BusSelector  OutputSignals=RemoteControl_dem.brake_dem
  Bus Selector8 : BusSelector  OutputSignals=MOTOR.MOTOR1.MCU2,MOTOR.MOTOR3.MCU2-2,MOTOR.MOTOR5.MCU2_4,MOTOR.MOTOR2.MCU2_1,MOTOR.MOTOR4.MCU2_3,MOTOR.MOTOR6.MCU2_5
  Constant1 : Constant  Value=bratrq_max  OutDataTypeStr=single  SampleTime=-1
  Constant2 : Constant  Value=0  OutDataTypeStr=single  SampleTime=-1
  Constant3 : Constant  Value=0  OutDataTypeStr=single  SampleTime=-1
  Constant4 : Constant  Value=0  OutDataTypeStr=single  SampleTime=-1
  Gain4 : Gain  Gain=1/2  OutDataTypeStr=single
  Gain5 : Gain  Gain=1/100  OutDataTypeStr=single
  Gain6 : Gain  Gain=1/2  OutDataTypeStr=single
  Gain7 : Gain  Gain=1/2  OutDataTypeStr=single
  HeartBeat : MATLAB Function  TreatAsAtomicUnit=on
  HeartBeat1 : MATLAB Function  TreatAsAtomicUnit=on
  HeartBeat2 : MATLAB Function  TreatAsAtomicUnit=on
  HeartBeat3 : MATLAB Function  TreatAsAtomicUnit=on
  HeartBeat4 : MATLAB Function  TreatAsAtomicUnit=on
  HeartBeat5 : MATLAB Function  TreatAsAtomicUnit=on
  Memory{,1..4,6} (6 alike) : Memory  InheritSampleTime=on
  Mux{,1..5} (6 alike) : Mux  Inputs=6
  Product : Product
  Saturation{,1..3,8..9} (6 alike) : Saturate  UpperLimit=trqmax_yd  LowerLimit=0  OutDataTypeStr=single
  Saturation10 : Saturate  UpperLimit=zhuanxiang_up  LowerLimit=zhuanxiang_down
  Saturation11 : Saturate  UpperLimit=zhuanxiang_up  LowerLimit=zhuanxiang_down
  Saturation12 : Saturate  UpperLimit=zhuanxiang_up  LowerLimit=zhuanxiang_down
  Saturation13 : Saturate  UpperLimit=zhidong_up  LowerLimit=zhidong_down
  Saturation6 : Saturate  UpperLimit=premax  LowerLimit=0  OutDataTypeStr=single
  Saturation7 : Saturate  UpperLimit=premax  LowerLimit=0  OutDataTypeStr=single
  SpdSet_dem{,1..5} (6 alike) : Constant  OutDataTypeStr=single  SampleTime=-1
  Subsystem : Subsystem
  Subsystem1 : Subsystem
  Subsystem2 : Subsystem
  Subsystem3 : Subsystem
  Subsystem4 : Subsystem
  Subsystem5 : Subsystem
  Switch{,1..4,6} (6 alike) : Switch  Criteria=u2 > Threshold
  Terminator : Terminator
  Terminator1 : Terminator
  Terminator2 : Terminator
  mot_enable{1..6} (6 alike) : Constant  OutDataTypeStr=single  SampleTime=-1
  mot_gear{,2,4,6,8,10} (6 alike) : Constant  Value=2  OutDataTypeStr=single  SampleTime=-1
  mot_gear{1,3,5,7,9,11} (6 alike) : Constant  OutDataTypeStr=single  SampleTime=-1
  mot_mode{,1..5} (6 alike) : Constant  Value=0  OutDataTypeStr=single  SampleTime=-1
  容错控制 : Subsystem
  左右侧电机分配及功率限制 : Subsystem
  mot_lf : Outport
  mot_lm : Outport  Port=2
  mot_lr : Outport  Port=3
  mot_rf : Outport  Port=4
  mot_rm : Outport  Port=5
  mot_rr : Outport  Port=6
  motec_position_1 : Outport  Port=7
  motec_position_2 : Outport  Port=8
  motec_position_3 : Outport  Port=9
  motec_position_4 : Outport  Port=10
  wires:
  Signals/1 -> [Signals], Bus Selector5/1
  左右侧电机分配及功率限制/2(trq_dem_r) -> 容错控制/2(trq_dem_r)
  左右侧电机分配及功率限制/1(trq_dem_l) -> 容错控制/1(trq_dem_l)
  左右侧电机分配及功率限制/6(trqlim_rf) -> 容错控制/6(trqlim_rf)
  左右侧电机分配及功率限制/5(trqlim_lr) -> 容错控制/5(trqlim_lr)
  左右侧电机分配及功率限制/8(trqlim_rr) -> 容错控制/8(trqlim_rr)
  左右侧电机分配及功率限制/3(trqlim_lf) -> 容错控制/3(trqlim_lf)
  容错控制/1(trq_dem_lf) -> [trq_dem_lf]
  容错控制/4(trq_dem_rf) -> [trq_dem_rf]
  容错控制/6(trq_dem_rr) -> [trq_dem_rr]
  容错控制/7(bra_pre_l) -> [bra_pre_l]
  容错控制/8(bra_pre_r) -> [bra_pre_r]
  容错控制/3(trq_dem_lr) -> [trq_dem_lr]
  Switch/1 -> Mux/3
  mot_mode/1 -> Mux/2
  [trq_dem_lf] -> Saturation/1
  Saturation/1 -> Mux/5
  Mux/1 -> mot_lf/1
  HeartBeat/1(life) -> Mux/6, Memory/1
  Memory/1 -> HeartBeat/1(life_pre)
  容错控制/9(mode) -> Terminator/1
  [steer_dem] -> Switch/2
  mot_gear1/1 -> Switch/3
  mot_gear/1 -> Switch/1
  [Signals] -> Bus Selector7/1
  1-D Lookup Table3/1 -> Saturation7/1
  Constant1/1 -> Product/1
  Bus Selector7/1 -> 容错控制/17(brake_dem), Gain5/1  "<brake_dem>"
  Product/1 -> Gain4/1
  Gain4/1 -> Gain7/1, Gain6/1
  Gain5/1 -> Product/2
  Gain6/1 -> 1-D Lookup Table3/1
  Gain7/1 -> 1-D Lookup Table1/1
  1-D Lookup Table1/1 -> Saturation6/1
  Saturation7/1 -> 容错控制/15(bra_dem_l)
  Saturation6/1 -> 容错控制/16(bra_dem_r)
  Bus Selector5/14 -> 左右侧电机分配及功率限制/14(TrqLimU_dig_rf)  "<MCU0_1TorqueMax>"
  Bus Selector5/13 -> 左右侧电机分配及功率限制/13(TrqLimU_dig_lr)  "<MCU0_4TorqueMax>"
  Bus Selector5/16 -> 左右侧电机分配及功率限制/16(TrqLimU_dig_rr)  "<MCU0_5TorqueMax>"
  Bus Selector5/12 -> 左右侧电机分配及功率限制/12(TrqLimU_dig_lm)  "<MCU0_2TorqueMax>"
  Bus Selector5/15 -> 左右侧电机分配及功率限制/15(TrqLimU_dig_rm)  "<MCU0_3TorqueMax>"
  Bus Selector5/1 -> [steer_dem], 左右侧电机分配及功率限制/1(steer_dem)  "<steer_dem>"
  Bus Selector5/3 -> 左右侧电机分配及功率限制/3(pwr_dis_bat1)  "<BMS5_1_15s_InstanceDisPower>"
  Bus Selector5/4 -> 左右侧电机分配及功率限制/4(pwr_dis_bat2)  "<BMS5_2_15s_InstanceDisPower>"
  Bus Selector5/2 -> 左右侧电机分配及功率限制/2(pwr_dis_bat)  "<BMS5_15s_InstanceDisPower>"
  Bus Selector5/5 -> Abs/1  "<MCU0_SpeedFdk>"
  Bus Selector5/7 -> Abs2/1  "<MCU0_4SpeedFdk>"
  Bus Selector5/6 -> Abs1/1  "<MCU0_2SpeedFdk>"
  Bus Selector5/11 -> 左右侧电机分配及功率限制/11(TrqLimU_dig_lf)  "<MCU0_TorqueMax>"
  Bus Selector5/8 -> Abs3/1  "<MCU0_1SpeedFdk>"
  Bus Selector5/10 -> Abs5/1  "<MCU0_5SpeedFdk>"
  Bus Selector5/9 -> Abs4/1  "<MCU0_3SpeedFdk>"
  Abs/1 -> 左右侧电机分配及功率限制/5(speed_act_lf)
  Abs1/1 -> 左右侧电机分配及功率限制/6(speed_act_lm)
  Abs2/1 -> 左右侧电机分配及功率限制/7(speed_act_lr)
  Abs3/1 -> 左右侧电机分配及功率限制/8(speed_act_rf)
  Abs4/1 -> 左右侧电机分配及功率限制/9(speed_act_rm)
  Abs5/1 -> 左右侧电机分配及功率限制/10(speed_act_rr)
  左右侧电机分配及功率限制/4(trqlim_lm) -> 容错控制/4(trqlim_lm)
  左右侧电机分配及功率限制/7(trqlim_rm) -> 容错控制/7(trqlim_rm)
  [Signals] -> Bus Selector8/1
  Bus Selector8/1 -> Subsystem/1(MCU2)  "<MCU2>"
  Subsystem/1(guzhang_lf) -> 容错控制/9(guzhang_lf)
  Bus Selector8/2 -> Subsystem1/1(MCU2_2)  "<MCU2-2>"
  Subsystem1/1(guzhang_lm) -> 容错控制/10(guzhang_lm)
  Bus Selector8/3 -> Subsystem2/1(MCU2_4)  "<MCU2_4>"
  Subsystem2/1(guzhang_lr) -> 容错控制/11(guzhang_lr)
  Bus Selector8/4 -> Subsystem3/1(MCU2_1)  "<MCU2_1>"
  Subsystem3/1(guzhang_rf) -> 容错控制/12(guzhang_rf)
  Bus Selector8/5 -> Subsystem4/1(MCU2_3)  "<MCU2_3>"
  Subsystem4/1(guzhang_rm) -> 容错控制/13(guzhang_rm)
  Bus Selector8/6 -> Subsystem5/1(MCU2_5)  "<MCU2_5>"
  Subsystem5/1(guzhang_rr) -> 容错控制/14(guzhang_rr)
  容错控制/2(trq_dem_lm) -> [trq_dem_lm]
  容错控制/5(trq_dem_rm) -> [trq_dem_rm]
  mot_enable4/1 -> Mux/1
  SpdSet_dem/1 -> Mux/4
  Switch2/1 -> Mux2/3
  mot_mode2/1 -> Mux2/2
  [trq_dem_rf] -> Saturation2/1
  Saturation2/1 -> Mux2/5
  Mux2/1 -> mot_rf/1
  HeartBeat2/1(life) -> Memory3/1, Mux2/6
  Memory3/1 -> HeartBeat2/1(life_pre)
  [steer_dem] -> Switch2/2
  mot_gear3/1 -> Switch2/3
  mot_gear2/1 -> Switch2/1
  mot_enable2/1 -> Mux2/1
  SpdSet_dem1/1 -> Mux2/4
  Switch4/1 -> Mux4/3
  mot_mode4/1 -> Mux4/2
  [trq_dem_lm] -> Saturation8/1
  Saturation8/1 -> Mux4/5
  Mux4/1 -> mot_lm/1
  HeartBeat3/1(life) -> Memory4/1, Mux4/6
  Memory4/1 -> HeartBeat3/1(life_pre)
  [steer_dem] -> Switch4/2
  mot_gear5/1 -> Switch4/3
  mot_gear4/1 -> Switch4/1
  mot_enable6/1 -> Mux4/1
  SpdSet_dem4/1 -> Mux4/4
  Switch6/1 -> Mux5/3
  mot_mode5/1 -> Mux5/2
  [trq_dem_rm] -> Saturation9/1
  Saturation9/1 -> Mux5/5
  Mux5/1 -> mot_rm/1
  HeartBeat4/1(life) -> Mux5/6, Memory6/1
  Memory6/1 -> HeartBeat4/1(life_pre)
  [steer_dem] -> Switch6/2
  mot_gear7/1 -> Switch6/3
  mot_gear6/1 -> Switch6/1
  mot_enable5/1 -> Mux5/1
  SpdSet_dem5/1 -> Mux5/4
  Switch1/1 -> Mux1/3
  mot_mode1/1 -> Mux1/2
  [trq_dem_lr] -> Saturation1/1
  Saturation1/1 -> Mux1/5
  Mux1/1 -> mot_lr/1
  HeartBeat1/1(life) -> Memory1/1, Mux1/6
  Memory1/1 -> HeartBeat1/1(life_pre)
  [steer_dem] -> Switch1/2
  mot_gear9/1 -> Switch1/3
  mot_gear8/1 -> Switch1/1
  mot_enable1/1 -> Mux1/1
  SpdSet_dem2/1 -> Mux1/4
  Switch3/1 -> Mux3/3
  mot_mode3/1 -> Mux3/2
  [trq_dem_rr] -> Saturation3/1
  Saturation3/1 -> Mux3/5
  Mux3/1 -> mot_rr/1
  HeartBeat5/1(life) -> Mux3/6, Memory2/1
  Memory2/1 -> HeartBeat5/1(life_pre)
  [steer_dem] -> Switch3/2
  mot_gear11/1 -> Switch3/3
  mot_gear10/1 -> Switch3/1
  mot_enable3/1 -> Mux3/1
  SpdSet_dem3/1 -> Mux3/4
  1-D Lookup Table2/1 -> Saturation13/1
  [Signals] -> Bus Selector/1
  Constant3/1 -> Saturation12/1
  Saturation10/1 -> motec_position_1/1
  Saturation11/1 -> motec_position_2/1
  Saturation12/1 -> motec_position_3/1
  Saturation13/1 -> motec_position_4/1
  Bus Selector/1 -> 1-D Lookup Table2/1  "<brake_dem>"
  Constant2/1 -> Saturation10/1
  Constant4/1 -> Saturation11/1
  [bra_pre_l] -> Terminator1/1
  [bra_pre_r] -> Terminator2/1

== matlab function six_plus_six_AcmsteeringV09_main/MainControl/mode_control/backward/backward/Drive/驱动防滑控制TCS/直行TCS/直行/MATLAB Function5 ==
  data: TCS_switch input; flag_lf1 output; flag_lm1 output; flag_lf input; flag_lm input; flag_lr input; flag_lr1 output; flag_rf input; flag_rm input; flag_rr input; flag_rf1 output; flag_rm1 output; flag_rr1 output
 function [flag_lf1,flag_lm1,flag_lr1,flag_rf1,flag_rm1,flag_rr1] = fcn(TCS_switch,flag_lf,flag_lm,flag_lr,flag_rf,flag_rm,flag_rr)
%#codegen
if TCS_switch==0
    flag_lf1=single(0);
    flag_lm1=single(0);
    flag_lr1=single(0);
    flag_rf1=single(0);
    flag_rm1=single(0);
    flag_rr1=single(0);
else
    flag_lf1=single(flag_lf);
    flag_lm1=single(flag_lm);
    flag_lr1=single(flag_lr);
    flag_rf1=single(flag_rf);
    flag_rm1=single(flag_rm);
    flag_rr1=single(flag_rr);
end
end

== matlab function six_plus_six_AcmsteeringV09_main/Data_input/9/Enabled Subsystem/MATLAB Function1 ==
  data: data1 input; y output; data2 input; data3 input; data4 input
function y = fcn(data1,data2,data3,data4)
%#codegen
y1=data4*256^3+data3*256^2+data2*256+data1;
% y=typecast(uint32(y1),'single');
y=single(y1*10^-7);
end
% y = u;

== matlab function six_plus_six_AcmsteeringV09_main/MainControl/mode_control/backward/backward/Drive/MATLAB Function ==
  data: acc_y input; y output; ag_thr input
function y = fcn(acc_y,ag_thr)
%#codegen
if abs(acc_y)>=ag_thr
    y=int8(0);
else 
    y=int8(1);
end
end

== matlab function six_plus_six_AcmsteeringV09_main/MainControl/mode_control/Park/park/HeartBeat4 ==
  data: life_pre input; life output
function life = fcn(life_pre)
%#codegen
life=single(life_pre+1);
if life>255
    life=single(0);
end
end
